simulink library "lib_Convection_FilmCoolTref"  (R2015a)
settings: Solver=ode45  StartTime=0.0  StopTime=10.0  RelTol=1e-3
settings Model: Creator=jlkratz  LastModifiedBy=jlkratz

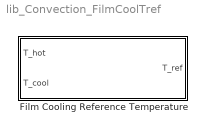
== system lib_Convection_FilmCoolTref ==
  Film Cooling Reference Temperature : Subsystem  mask(Film Cooling Reference Temperature){eta_M=0.5}
      mask prompts: eta_M "eta_M - film cooling coefficient"
      mask help: This function computes the effective temperature of the fluid on the surface of a structure due to film cooling. The model utilizes a film cooling coefficient to determine this reference temperature (T_ref) based one the temperatures of the hot flow path (T_hot) and cooling flow (T_cool). Units of the inputs must be consistent and the output will be in the same units as the input.
      mask Help: web(which('Convection_TSAT_FilmCoolTref.html'),'-helpbrowser')

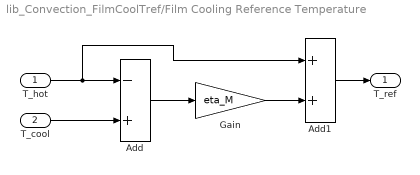
== system lib_Convection_FilmCoolTref/Film Cooling Reference Temperature ==
  T_hot : Inport
  T_cool : Inport  Port=2
  Add : Sum  Inputs=-+
  Add1 : Sum
  Gain : Gain  Gain=eta_M
  T_ref : Outport
  wires:
  T_cool/1 -> Add/2
  Add/1 -> Gain/1
  T_hot/1 -> Add/1, Add1/1
  Add1/1 -> T_ref/1
  Gain/1 -> Add1/2
